simulink model "leadlag_compensator"  (R2016a)
settings: Solver=VariableStepAuto  StartTime=0.0  StopTime=10.0  RelTol=1e-3
undefined symbols (not defined in the file): w_p, w_z
settings Model: Creator=rtw141  LastModifiedBy=rtw141
settings GRTTargetCC: GeneratePreprocessorConditionals=Use local settings

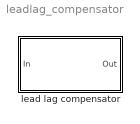
== system leadlag_compensator ==
  lead lag compensator : Subsystem

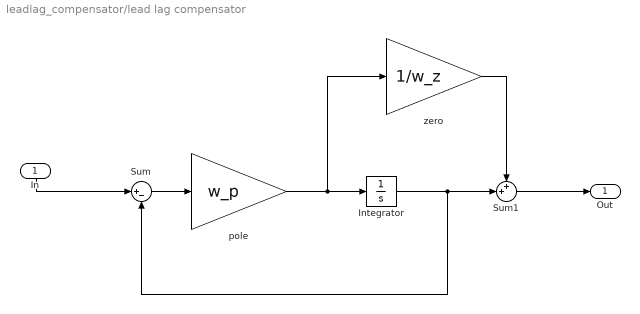
== system leadlag_compensator/lead lag compensator ==
  In : Inport
  Integrator : Integrator
  Sum : Sum  Inputs=|+-
  Sum1 : Sum  Inputs=++|
  pole : Gain  Gain=w_p
  zero : Gain  Gain=1/w_z
  Out : Outport
  wires:
  Sum1/1 -> Out/1
  pole/1 -> zero/1, Integrator/1
  Sum/1 -> pole/1
  Integrator/1 -> Sum1/2, Sum/2
  zero/1 -> Sum1/1
  In/1 -> Sum/1
